simulink model "trackingSFun"  (R2018b)
settings: Solver=FixedStepAuto  StartTime=0.0  StopTime=141  FixedStep=0.02  MaxStep=0.02  RelTol=1e-3  EnableMultiTasking=on
StopFcn:
  | track_erg=[tout,yout];
  | clear tout yout
libraries: simulink x1
settings Model: Creator=mkrug  LastModifiedBy=Reichl
settings DataIOCC: LimitDataPoints=on  MaxDataPoints=10000  SaveFormat=Array
settings OptimizationCC: BlockReduction=off  OptimizeBlockIOStorage=off  BufferReuse=off  GlobalBufferReuse=off  ExpressionFolding=off  LocalBlockOutputs=off  LifeSpan=inf  OptimizeDataStoreBuffers=off  BusAssignmentInplaceUpdate=off
settings DebuggingCC: SolverPrmCheckMsg=warning  AllowSymbolicDim=off  SFUnexpectedBacktrackingDiag=warning  SFNoUnconditionalDefaultTransitionDiag=warning  SFExecutionAtInitializationDiag=none
settings HardwareCC: ProdBitPerPointer=32  ProdBitPerSizeT=32  ProdBitPerPtrDiffT=32  ProdLargestAtomicFloat=None  ProdIntDivRoundTo=Undefined  ProdEndianess=Unspecified  ProdWordSize=32  ProdHWDeviceType=32-bit Generic
settings ModelReferenceCC: PropagateSignalLabelsOutOfModel=off
settings SFSimCC: SimUseLocalCustomCode=off
settings RTWCC: RTWUseLocalCustomCode=off
settings CodeAppCC: StateflowObjectComments=on
settings GRTTargetCC: TargetLangStandard=C89/C90 (ANSI)  GeneratePreprocessorConditionals=Disable all
settings ConfigComp: CovMetricSettings=dw  CovHtmlReporting=on  CovSaveCumulativeToWorkspaceVar=on  CovSaveSingleToWorkspaceVar=on  CovExternalEMLEnable=off  CovSFcnEnable=off

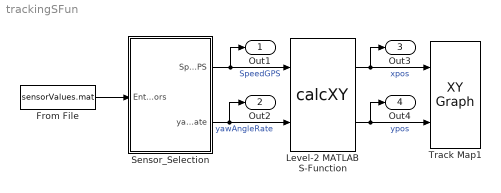
== system trackingSFun ==
  From File : FromFile  FileName=sensorValues.mat  SampleTime=0
  Level-2 MATLAB S-Function : M-S-Function  FunctionName=calcXY  Parameters=0, 0, 0
  Sensor_Selection : Subsystem
  Track Map1 : simulink/Sinks/XY Graph  xmin=-700  xmax=700  ymin=-700  ymax=700  st=-1
  Out1 : Outport
  Out2 : Outport  Port=2
  Out3 : Outport  Port=3
  Out4 : Outport  Port=4
  wires:
  From File/1 -> Sensor_Selection/1(EntireSensors)
  Sensor_Selection/2(yawAngleRate) -> Out2/1, Level-2 MATLAB S-Function/2  "yawAngleRate"
  Sensor_Selection/1(SpeedGPS) -> Out1/1, Level-2 MATLAB S-Function/1  "SpeedGPS"
  Level-2 MATLAB S-Function/1 -> Out3/1, Track Map1/1  "xpos"
  Level-2 MATLAB S-Function/2 -> Out4/1, Track Map1/2  "ypos"

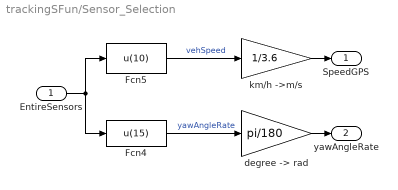
== system trackingSFun/Sensor_Selection ==
  EntireSensors : Inport
  Fcn4 : Fcn  Expr=u(15)
  Fcn5 : Fcn  Expr=u(10)
  "degree -> rad" : Gain  Gain=pi/180
  km/h ->m/s : Gain  Gain=1/3.6
  SpeedGPS : Outport
  yawAngleRate : Outport  Port=2
  wires:
  EntireSensors/1 -> Fcn5/1, Fcn4/1
  Fcn4/1 -> "degree -> rad"/1  "yawAngleRate"
  Fcn5/1 -> km/h ->m/s/1  "vehSpeed"
  km/h ->m/s/1 -> SpeedGPS/1
  "degree -> rad"/1 -> yawAngleRate/1
